simulink model "ztransform"  (R2024a)
settings: Solver=VariableStepAuto  StartTime=0.0  StopTime=10.0  RelTol=1e-3
settings Model: Creator=tusha  LastModifiedBy=tusha

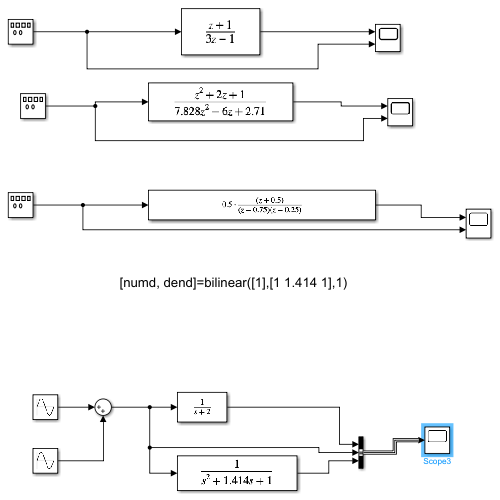
[thumbnail: Simulink's stored preview of the top-level diagram]
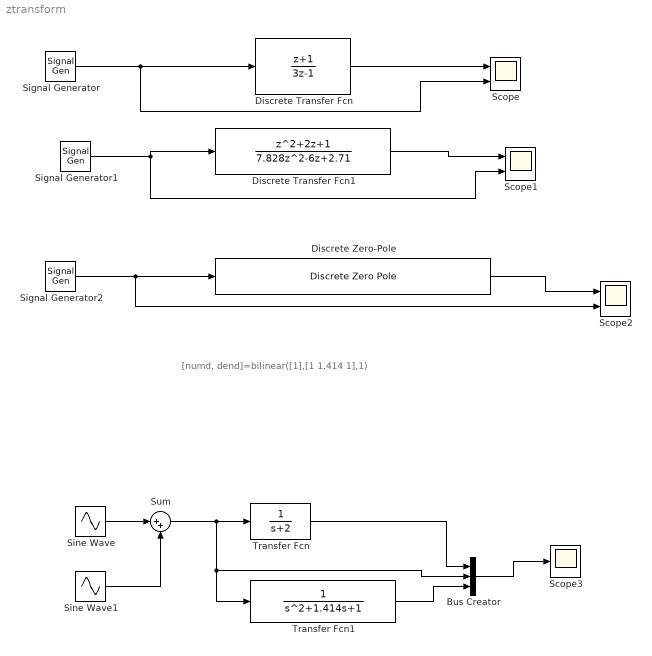
== system ztransform ==
  note: [numd, dend]=bilinear([1],[1 1.414 1],1)
  Bus Creator : BusCreator  Inputs=3
  Discrete Transfer Fcn : DiscreteTransferFcn  Numerator=[1 1]  Denominator=[3 -1]
  Discrete Transfer Fcn1 : DiscreteTransferFcn  Numerator=[1 2 1]  Denominator=[7.828 -6 2.71]
  Discrete Zero-Pole : DiscreteZeroPole  Zeros=[-0.5]  Poles=[0.75 0.25]  Gain=0.5  SampleTime=-1
  Scope : Scope  NumInputPorts=2
  Scope1 : Scope  NumInputPorts=2
  Scope2 : Scope  NumInputPorts=2
  Scope3 : Scope
  Signal Generator : SignalGenerator  Units=rad/sec
  Signal Generator1 : SignalGenerator  Units=rad/sec
  Signal Generator2 : SignalGenerator  Units=rad/sec
  Sine Wave : Sin  SampleTime=0
  Sine Wave1 : Sin  Frequency=10  SampleTime=0
  Sum : Sum  Inputs=|++
  Transfer Fcn : TransferFcn  Denominator=[1 2]
  Transfer Fcn1 : TransferFcn  Denominator=[1 1.414 1]
  wires:
  Signal Generator/1 -> Scope/2, Discrete Transfer Fcn/1
  Discrete Transfer Fcn/1 -> Scope/1
  Signal Generator1/1 -> Scope1/2, Discrete Transfer Fcn1/1
  Discrete Transfer Fcn1/1 -> Scope1/1
  Signal Generator2/1 -> Scope2/2, Discrete Zero-Pole/1
  Discrete Zero-Pole/1 -> Scope2/1
  Bus Creator/1 -> Scope3/1
  Sine Wave/1 -> Sum/1
  Sine Wave1/1 -> Sum/2
  Sum/1 -> Bus Creator/2, Transfer Fcn1/1, Transfer Fcn/1
  Transfer Fcn1/1 -> Bus Creator/3
  Transfer Fcn/1 -> Bus Creator/1
